simulink model "v14_shiftreg_prs"  (R2019b)
settings: Solver=FixedStepAuto  StartTime=0.0  StopTime=100  FixedStep=1  MaxStep=1  RelTol=1e-3
libraries: simulink_extras x1
settings Model: Creator=MARAT  LastModifiedBy=Marat
settings SFSimCC: CustomCodeUndefinedFunction=UseInterfaceOnly

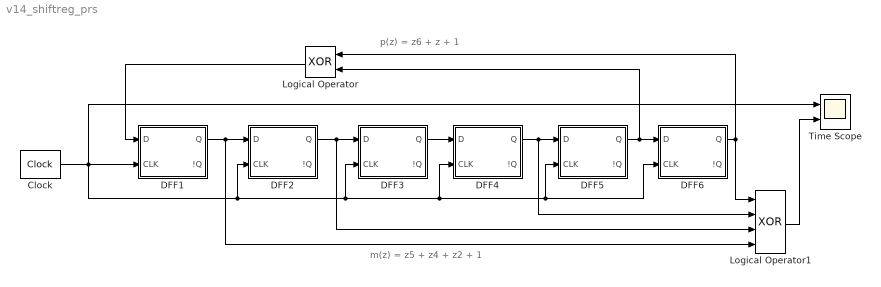
== system v14_shiftreg_prs ==
  note: m(z) = z5 + z4 + z2 + 1
  note: p(z) = z6 + z + 1
  Clock : simulink_extras/Flip Flops/Clock  period=2
  DFF1 : Subsystem  mask{intstate=0}
      mask prompts: intstate "Initial State"
      mask init:
      | dint = intstate;
      mask Display: disp(['Q = ' int2str(dint)])
  DFF2 : Subsystem  mask{intstate=0}
      mask prompts: intstate "Initial State"
      mask init:
      | dint = intstate;
      mask Display: disp(['Q = ' int2str(dint)])
  DFF3 : Subsystem  mask{intstate=1}
      mask prompts: intstate "Initial State"
      mask init:
      | dint = intstate;
      mask Display: disp(['Q = ' int2str(dint)])
  DFF4 : Subsystem  mask{intstate=0}
      mask prompts: intstate "Initial State"
      mask init:
      | dint = intstate;
      mask Display: disp(['Q = ' int2str(dint)])
  DFF5 : Subsystem  mask{intstate=1}
      mask prompts: intstate "Initial State"
      mask init:
      | dint = intstate;
      mask Display: disp(['Q = ' int2str(dint)])
  DFF6 : Subsystem  mask{intstate=1}
      mask prompts: intstate "Initial State"
      mask init:
      | dint = intstate;
      mask Display: disp(['Q = ' int2str(dint)])
  Logical Operator : Logic  Operator=XOR  AllPortsSameDT=off  OutDataTypeStr=boolean
  Logical Operator1 : Logic  Operator=XOR  Inputs=4  AllPortsSameDT=off  OutDataTypeStr=boolean
  Time Scope : Scope  NumInputPorts=2
  wires:
  Logical Operator1/1 -> Time Scope/2
  DFF6/1(Q) -> Logical Operator1/1, Logical Operator/1
  DFF4/1(Q) -> DFF5/1(D), Logical Operator1/2
  DFF2/1(Q) -> DFF3/1(D), Logical Operator1/3
  Logical Operator/1 -> DFF1/1(D)
  DFF1/1(Q) -> DFF2/1(D), Logical Operator1/4
  DFF3/1(Q) -> DFF4/1(D)
  DFF5/1(Q) -> DFF6/1(D), Logical Operator/2
  Clock/1 -> Time Scope/1, DFF2/2(CLK), DFF3/2(CLK), DFF4/2(CLK), DFF6/2(CLK), DFF5/2(CLK), DFF1/2(CLK)

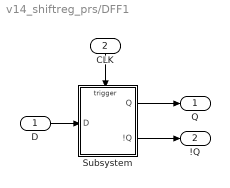
== system v14_shiftreg_prs/DFF1 ==
  D : Inport
  CLK : Inport  Port=2
  Subsystem : Subsystem
  Q : Outport  InitialOutput=0  VectorParamsAs1DForOutWhenUnconnected=off
  !Q : Outport  Port=2  InitialOutput=1  VectorParamsAs1DForOutWhenUnconnected=off
  wires:
  CLK/1 -> Subsystem/Trigger
  D/1 -> Subsystem/1(D)
  Subsystem/1(Q) -> Q/1
  Subsystem/2(!Q) -> !Q/1

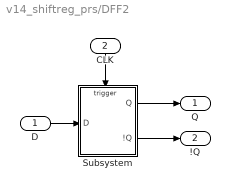
== system v14_shiftreg_prs/DFF2 ==
  D : Inport
  CLK : Inport  Port=2
  Subsystem : Subsystem
  Q : Outport  InitialOutput=0  VectorParamsAs1DForOutWhenUnconnected=off
  !Q : Outport  Port=2  InitialOutput=1  VectorParamsAs1DForOutWhenUnconnected=off
  wires:
  Subsystem/2(!Q) -> !Q/1
  Subsystem/1(Q) -> Q/1
  D/1 -> Subsystem/1(D)
  CLK/1 -> Subsystem/Trigger

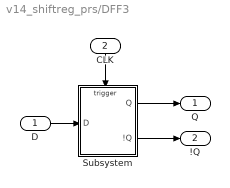
== system v14_shiftreg_prs/DFF3 ==
  D : Inport
  CLK : Inport  Port=2
  Subsystem : Subsystem
  Q : Outport  InitialOutput=0  VectorParamsAs1DForOutWhenUnconnected=off
  !Q : Outport  Port=2  InitialOutput=1  VectorParamsAs1DForOutWhenUnconnected=off
  wires:
  CLK/1 -> Subsystem/Trigger
  D/1 -> Subsystem/1(D)
  Subsystem/1(Q) -> Q/1
  Subsystem/2(!Q) -> !Q/1

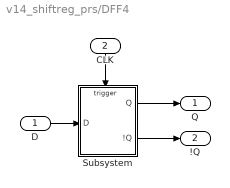
== system v14_shiftreg_prs/DFF4 ==
  D : Inport
  CLK : Inport  Port=2
  Subsystem : Subsystem
  Q : Outport  InitialOutput=0  VectorParamsAs1DForOutWhenUnconnected=off
  !Q : Outport  Port=2  InitialOutput=1  VectorParamsAs1DForOutWhenUnconnected=off
  wires:
  Subsystem/2(!Q) -> !Q/1
  Subsystem/1(Q) -> Q/1
  D/1 -> Subsystem/1(D)
  CLK/1 -> Subsystem/Trigger

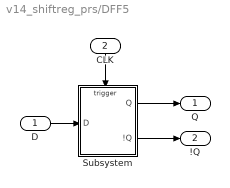
== system v14_shiftreg_prs/DFF5 ==
  D : Inport
  CLK : Inport  Port=2
  Subsystem : Subsystem
  Q : Outport  InitialOutput=0  VectorParamsAs1DForOutWhenUnconnected=off
  !Q : Outport  Port=2  InitialOutput=1  VectorParamsAs1DForOutWhenUnconnected=off
  wires:
  CLK/1 -> Subsystem/Trigger
  D/1 -> Subsystem/1(D)
  Subsystem/1(Q) -> Q/1
  Subsystem/2(!Q) -> !Q/1

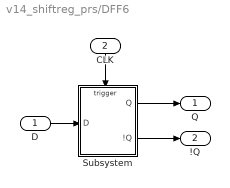
== system v14_shiftreg_prs/DFF6 ==
  D : Inport
  CLK : Inport  Port=2
  Subsystem : Subsystem
  Q : Outport  InitialOutput=0  VectorParamsAs1DForOutWhenUnconnected=off
  !Q : Outport  Port=2  InitialOutput=1  VectorParamsAs1DForOutWhenUnconnected=off
  wires:
  Subsystem/2(!Q) -> !Q/1
  Subsystem/1(Q) -> Q/1
  D/1 -> Subsystem/1(D)
  CLK/1 -> Subsystem/Trigger

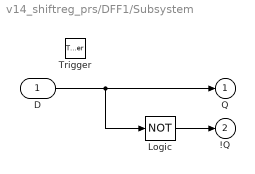
== system v14_shiftreg_prs/DFF1/Subsystem ==
  D : Inport  LatchByDelayingOutsideSignal=on
  Trigger : TriggerPort  VariantControl=Variant  StatesWhenEnabling=reset
  Logic : Logic  Operator=NOT  Inputs=1
  Q : Outport  OutputWhenDisabled=reset  InitialOutput=intstate > 0  VectorParamsAs1DForOutWhenUnconnected=off
  !Q : Outport  Port=2  OutputWhenDisabled=reset  InitialOutput=intstate < 1  VectorParamsAs1DForOutWhenUnconnected=off
  wires:
  Logic/1 -> !Q/1
  D/1 -> Q/1, Logic/1

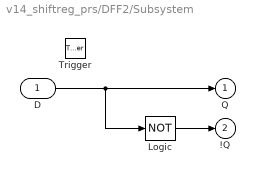
== system v14_shiftreg_prs/DFF2/Subsystem ==
  D : Inport  LatchByDelayingOutsideSignal=on
  Trigger : TriggerPort  VariantControl=Variant  StatesWhenEnabling=reset
  Logic : Logic  Operator=NOT  Inputs=1
  Q : Outport  OutputWhenDisabled=reset  InitialOutput=intstate > 0  VectorParamsAs1DForOutWhenUnconnected=off
  !Q : Outport  Port=2  OutputWhenDisabled=reset  InitialOutput=intstate < 1  VectorParamsAs1DForOutWhenUnconnected=off
  wires:
  D/1 -> Logic/1, Q/1
  Logic/1 -> !Q/1

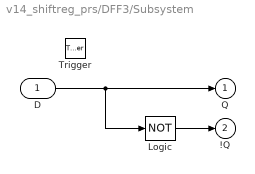
== system v14_shiftreg_prs/DFF3/Subsystem ==
  D : Inport  LatchByDelayingOutsideSignal=on
  Trigger : TriggerPort  VariantControl=Variant  StatesWhenEnabling=reset
  Logic : Logic  Operator=NOT  Inputs=1
  Q : Outport  OutputWhenDisabled=reset  InitialOutput=intstate > 0  VectorParamsAs1DForOutWhenUnconnected=off
  !Q : Outport  Port=2  OutputWhenDisabled=reset  InitialOutput=intstate < 1  VectorParamsAs1DForOutWhenUnconnected=off
  wires:
  Logic/1 -> !Q/1
  D/1 -> Q/1, Logic/1

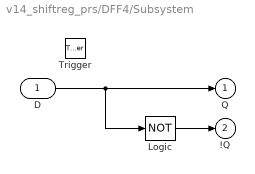
== system v14_shiftreg_prs/DFF4/Subsystem ==
  D : Inport  LatchByDelayingOutsideSignal=on
  Trigger : TriggerPort  VariantControl=Variant  StatesWhenEnabling=reset
  Logic : Logic  Operator=NOT  Inputs=1
  Q : Outport  OutputWhenDisabled=reset  InitialOutput=intstate > 0  VectorParamsAs1DForOutWhenUnconnected=off
  !Q : Outport  Port=2  OutputWhenDisabled=reset  InitialOutput=intstate < 1  VectorParamsAs1DForOutWhenUnconnected=off
  wires:
  D/1 -> Logic/1, Q/1
  Logic/1 -> !Q/1

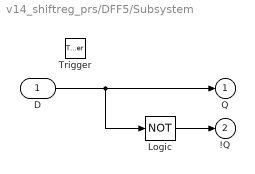
== system v14_shiftreg_prs/DFF5/Subsystem ==
  D : Inport  LatchByDelayingOutsideSignal=on
  Trigger : TriggerPort  VariantControl=Variant  StatesWhenEnabling=reset
  Logic : Logic  Operator=NOT  Inputs=1
  Q : Outport  OutputWhenDisabled=reset  InitialOutput=intstate > 0  VectorParamsAs1DForOutWhenUnconnected=off
  !Q : Outport  Port=2  OutputWhenDisabled=reset  InitialOutput=intstate < 1  VectorParamsAs1DForOutWhenUnconnected=off
  wires:
  Logic/1 -> !Q/1
  D/1 -> Q/1, Logic/1

== system v14_shiftreg_prs/DFF6/Subsystem ==
  D : Inport  LatchByDelayingOutsideSignal=on
  Trigger : TriggerPort  VariantControl=Variant  StatesWhenEnabling=reset
  Logic : Logic  Operator=NOT  Inputs=1
  Q : Outport  OutputWhenDisabled=reset  InitialOutput=intstate > 0  VectorParamsAs1DForOutWhenUnconnected=off
  !Q : Outport  Port=2  OutputWhenDisabled=reset  InitialOutput=intstate < 1  VectorParamsAs1DForOutWhenUnconnected=off
  wires:
  D/1 -> Logic/1, Q/1
  Logic/1 -> !Q/1
